simulink model "gps"  (Simulink 7.5)
settings: Solver=ode45  StartTime=0.0  StopTime=10.0  RelTol=1e-3
undefined symbols (not defined in the file or in its folder): magnitude, serial
libraries: dspsrcs4 x32, dspsigops x4, dsparch4 x3, dspstat3 x3, dspindex x3, instrumentlib x2, tiiqmathlib x1, dspxfrm3 x1
settings Model: Creator=sisa  LastModifiedBy=sisa

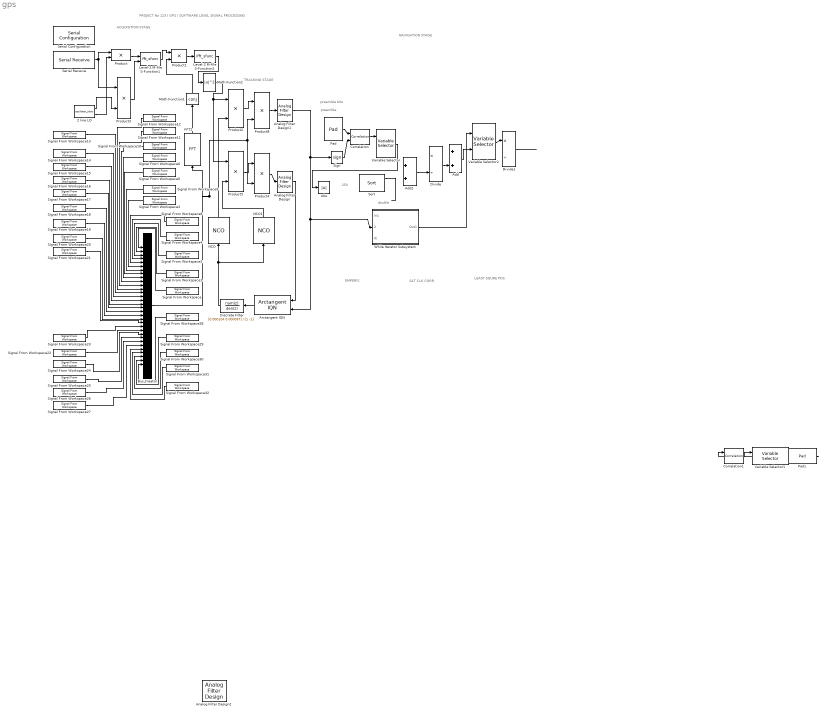
== system gps ==
  note: PROJECT No 123 ( GPS ) SOFTWARE LEVEL SIGNAL PROCESSING
  note: 253
  note: double
  note: preamble
  note: preamble bits
  note: ACQUISITION STAGE
  note: TRACKING STAGE
  note: EMPERIS
  note: NAVIGATION STAGE
  note: SAT CLK CORR
  note: LEAST SQURE POS
  2 line LO : M-S-Function  FunctionName=oscillator_sfunc  Parameters=1/38192000
  Abs : Abs  OutDataType=fixdt(1, 16)  OutScaling=2^0
  Add : Sum  OutDataType=fixdt(1, 16)  OutScaling=2^-10
  Add1 : Sum  OutDataType=fixdt(1, 16)  OutScaling=2^-10
  Analog Filter Design : dsparch4/Analog Filter Design  method=Butterworth  filttype=Lowpass  N=8  Wlo=30  Whi=80  Rp=2  Rs=40
  Analog Filter Design1 : dsparch4/Analog Filter Design  method=Chebyshev I  filttype=Lowpass  N=8  Wlo=30  Whi=80  Rp=2  Rs=40
  Analog Filter Design2 : dsparch4/Analog Filter Design  method=Butterworth  filttype=Lowpass  N=8  Wlo=30  Whi=80  Rp=2  Rs=40
  Arctangent IQN : tiiqmathlib/Arctangent IQN  tanOption=atan2PU (per unit)
  Bus Creator : BusCreator  Inputs=32  UseBusObject=on
  Correlation : dspstat3/Correlation  DialogController=dspDDGCreate  DialogControllerArgs=DataTag0  domain=Time  outputDataTypeStr=Inherit: Same as accumulator  outputLastDataTypeStr=Inherit: Same as accumulator  outputMin=[]  outputMax=[]  roundingMode=Floor  overflowMode=off
  Correlation1 : dspstat3/Correlation  DialogController=dspDDGCreate  DialogControllerArgs=DataTag1  domain=Time  outputDataTypeStr=Inherit: Same as accumulator  outputLastDataTypeStr=Inherit: Same as accumulator  outputMin=[]  outputMax=[]  roundingMode=Floor  overflowMode=off
  Discrete Filter : DiscreteFilter  Numerator=[0.000104 0.000097]  Denominator=[1 -1]  SampleTime=1
  Divide : Product  Inputs=*/  OutDataType=fixdt(1, 16)  OutScaling=2^-10
  Divide1 : Product  Inputs=*/  OutDataType=fixdt(1, 16)  OutScaling=2^-10
  FFT2 : dspxfrm3/FFT  DialogController=dspDDGCreate  DialogControllerArgs=DataTag2  CompMethod=Table lookup  TableOpt=NEW  TableOptActive=Speed  BitRevOrder=off  InheritFFTLength=on  FFTLength=64  SkipNorm=off  firstCoeffDataTypeStr=Inherit: Same word length as input  firstCoeffLastDataTypeStr=Inherit: Same word length as input  outputMin=[]  outputMax=[]  roundingMode=Floor  overflowMode=off
  Level-2 M-file S-Function1 : M-S-Function  FunctionName=fft_sfunc
  Level-2 M-file S-Function2 : M-S-Function  FunctionName=ifft_sfunc
  Math Function1 : Math  Operator=conj  OutputSignalType=complex  OutDataType=fixdt(1, 16)  OutScaling=2^0  SaturateOnIntegerOverflow=on
  Math Function2 : Math  Operator=magnitude^2  OutputSignalType=real  OutDataType=fixdt(1, 16)  OutScaling=2^0  SaturateOnIntegerOverflow=on
  NCO : dspsigops/NCO  DialogController=dspdialog.NCO  AccIncSrc=Input port  AccInc=100  PhaseOffsetSrc=Specify via dialog  PhaseOffset=0  AccumWL=16  HasDither=on  DitherWL=4  PNgeneratorLength=19  HasPhaseQuantizer=on  TableDepth=12  HasOutputPhaseError=off  Formula=Cosine  DataType=Binary point scaling  OutputWL=16  OutputFL=14  CompMethod=Table lookup (no interpolation)  SampleTime=1  SamplesPerFrame=1
  NCO1 : dspsigops/NCO  DialogController=dspdialog.NCO  AccIncSrc=Input port  AccInc=100  PhaseOffsetSrc=Specify via dialog  PhaseOffset=0  AccumWL=16  HasDither=on  DitherWL=4  PNgeneratorLength=19  HasPhaseQuantizer=on  TableDepth=12  HasOutputPhaseError=off  Formula=Sine  DataType=Binary point scaling  OutputWL=16  OutputFL=14  CompMethod=Table lookup (no interpolation)  SampleTime=1  SamplesPerFrame=1
  Pad : dspsigops/Pad  padAlong=Columns  dimsToPad=1  valSrc=Specify via dialog  padVal=0  spec=Output size  padNumOutRowsSpecMethod=User-specified  numOutRows=1  padNumOutColsSpecMethod=User-specified  numOutCols=1  isVarDimsMode=off  padBeginning=0  padEnd=0  outSizeMode=User-specified  outSize=1  padSigAt=End  trunc_flag=None  roundingMode=Floor  overflowMode=off  truncOrWrapMode=Truncate  wrap_flag=None
  Pad1 : dspsigops/Pad  padAlong=Columns  dimsToPad=1  valSrc=Specify via dialog  padVal=0  spec=Output size  padNumOutRowsSpecMethod=User-specified  numOutRows=1  padNumOutColsSpecMethod=User-specified  numOutCols=1  isVarDimsMode=off  padBeginning=0  padEnd=0  outSizeMode=User-specified  outSize=1  padSigAt=End  trunc_flag=None  roundingMode=Floor  overflowMode=off  truncOrWrapMode=Truncate  wrap_flag=None
  Product{,1..5,8} (7 alike) : Product  OutDataType=fixdt(1, 16)  OutScaling=2^0  RndMeth=Zero
  Serial Configuration : instrumentlib/Serial Configuration  Priority=-200000  DialogController=instrumentcreatedialog  DialogControllerArgs=DataTag3  ComPortMenu=COM1  ComPort=COM1  ObjConstructor=serial('COM1');  BaudRate=9600  DataBits=8  Parity=none  StopBits=1  FlowControl=none  Timeout=10  ByteOrder=LittleEndian
  Serial Receive : instrumentlib/Serial Receive  DialogController=instrumentcreatedialog  DialogControllerArgs=DataTag4  ComPortMenu=COM1  ComPort=COM1  ObjConstructor=serial('COM1');  Header=none  Terminator=<none>  DataSize="[1  1]"  DataType=uint8  EnableBlockingMode=on  ActionDataUnavailable=Output last received value  CustomValue=0  SampleTime=0.01
  Sign : Signum
  Signal From Workspace : dspsrcs4/Signal From Workspace  SystemSampleTime=-1  X=PN01  Ts=1  nsamps=1  OutputAfterFinalValue=Setting to zero  ignoreOrWarnInputAndFrameLengths=off
  Signal From Workspace1 : dspsrcs4/Signal From Workspace  SystemSampleTime=-1  X=PN02  Ts=1  nsamps=1  OutputAfterFinalValue=Setting to zero  ignoreOrWarnInputAndFrameLengths=off
  Signal From Workspace10 : dspsrcs4/Signal From Workspace  SystemSampleTime=-1  X=PN10  Ts=1  nsamps=1  OutputAfterFinalValue=Setting to zero  ignoreOrWarnInputAndFrameLengths=off
  Signal From Workspace11 : dspsrcs4/Signal From Workspace  SystemSampleTime=-1  X=PN11  Ts=1  nsamps=1  OutputAfterFinalValue=Setting to zero  ignoreOrWarnInputAndFrameLengths=off
  Signal From Workspace12 : dspsrcs4/Signal From Workspace  SystemSampleTime=-1  X=PN12  Ts=1  nsamps=1  OutputAfterFinalValue=Setting to zero  ignoreOrWarnInputAndFrameLengths=off
  Signal From Workspace13 : dspsrcs4/Signal From Workspace  SystemSampleTime=-1  X=PN13  Ts=1  nsamps=1  OutputAfterFinalValue=Setting to zero  ignoreOrWarnInputAndFrameLengths=off
  Signal From Workspace14 : dspsrcs4/Signal From Workspace  SystemSampleTime=-1  X=PN14  Ts=1  nsamps=1  OutputAfterFinalValue=Setting to zero  ignoreOrWarnInputAndFrameLengths=off
  Signal From Workspace15 : dspsrcs4/Signal From Workspace  SystemSampleTime=-1  X=PN15  Ts=1  nsamps=1  OutputAfterFinalValue=Setting to zero  ignoreOrWarnInputAndFrameLengths=off
  Signal From Workspace16 : dspsrcs4/Signal From Workspace  SystemSampleTime=-1  X=PN16  Ts=1  nsamps=1  OutputAfterFinalValue=Setting to zero  ignoreOrWarnInputAndFrameLengths=off
  Signal From Workspace17 : dspsrcs4/Signal From Workspace  SystemSampleTime=-1  X=PN17  Ts=1  nsamps=1  OutputAfterFinalValue=Setting to zero  ignoreOrWarnInputAndFrameLengths=off
  Signal From Workspace18 : dspsrcs4/Signal From Workspace  SystemSampleTime=-1  X=PN18  Ts=1  nsamps=1  OutputAfterFinalValue=Setting to zero  ignoreOrWarnInputAndFrameLengths=off
  Signal From Workspace19 : dspsrcs4/Signal From Workspace  SystemSampleTime=-1  X=PN19  Ts=1  nsamps=1  OutputAfterFinalValue=Setting to zero  ignoreOrWarnInputAndFrameLengths=off
  Signal From Workspace2 : dspsrcs4/Signal From Workspace  SystemSampleTime=-1  X=PN03  Ts=1  nsamps=1  OutputAfterFinalValue=Setting to zero  ignoreOrWarnInputAndFrameLengths=off
  Signal From Workspace20 : dspsrcs4/Signal From Workspace  SystemSampleTime=-1  X=PN20  Ts=1  nsamps=1  OutputAfterFinalValue=Setting to zero  ignoreOrWarnInputAndFrameLengths=off
  Signal From Workspace21 : dspsrcs4/Signal From Workspace  SystemSampleTime=-1  X=PN21  Ts=1  nsamps=1  OutputAfterFinalValue=Setting to zero  ignoreOrWarnInputAndFrameLengths=off
  Signal From Workspace22 : dspsrcs4/Signal From Workspace  SystemSampleTime=-1  X=PN23  Ts=1  nsamps=1  OutputAfterFinalValue=Setting to zero  ignoreOrWarnInputAndFrameLengths=off
  Signal From Workspace23 : dspsrcs4/Signal From Workspace  SystemSampleTime=-1  X=PN22  Ts=1  nsamps=1  OutputAfterFinalValue=Setting to zero  ignoreOrWarnInputAndFrameLengths=off
  Signal From Workspace24 : dspsrcs4/Signal From Workspace  SystemSampleTime=-1  X=PN24  Ts=1  nsamps=1  OutputAfterFinalValue=Setting to zero  ignoreOrWarnInputAndFrameLengths=off
  Signal From Workspace25 : dspsrcs4/Signal From Workspace  SystemSampleTime=-1  X=PN25  Ts=1  nsamps=1  OutputAfterFinalValue=Setting to zero  ignoreOrWarnInputAndFrameLengths=off
  Signal From Workspace26 : dspsrcs4/Signal From Workspace  SystemSampleTime=-1  X=PN26  Ts=1  nsamps=1  OutputAfterFinalValue=Setting to zero  ignoreOrWarnInputAndFrameLengths=off
  Signal From Workspace27 : dspsrcs4/Signal From Workspace  SystemSampleTime=-1  X=PN27  Ts=1  nsamps=1  OutputAfterFinalValue=Setting to zero  ignoreOrWarnInputAndFrameLengths=off
  Signal From Workspace28 : dspsrcs4/Signal From Workspace  SystemSampleTime=-1  X=PN28  Ts=1  nsamps=1  OutputAfterFinalValue=Setting to zero  ignoreOrWarnInputAndFrameLengths=off
  Signal From Workspace29 : dspsrcs4/Signal From Workspace  SystemSampleTime=-1  X=PN29  Ts=1  nsamps=1  OutputAfterFinalValue=Setting to zero  ignoreOrWarnInputAndFrameLengths=off
  Signal From Workspace3 : dspsrcs4/Signal From Workspace  SystemSampleTime=-1  X=PN06  Ts=1  nsamps=1  OutputAfterFinalValue=Setting to zero  ignoreOrWarnInputAndFrameLengths=off
  Signal From Workspace30 : dspsrcs4/Signal From Workspace  SystemSampleTime=-1  X=PN30  Ts=1  nsamps=1  OutputAfterFinalValue=Setting to zero  ignoreOrWarnInputAndFrameLengths=off
  Signal From Workspace31 : dspsrcs4/Signal From Workspace  SystemSampleTime=-1  X=PN31  Ts=1  nsamps=1  OutputAfterFinalValue=Setting to zero  ignoreOrWarnInputAndFrameLengths=off
  Signal From Workspace32 : dspsrcs4/Signal From Workspace  SystemSampleTime=-1  X=PN32  Ts=1  nsamps=1  OutputAfterFinalValue=Setting to zero  ignoreOrWarnInputAndFrameLengths=off
  Signal From Workspace4 : dspsrcs4/Signal From Workspace  SystemSampleTime=-1  X=PN04  Ts=1  nsamps=1  OutputAfterFinalValue=Setting to zero  ignoreOrWarnInputAndFrameLengths=off
  Signal From Workspace5 : dspsrcs4/Signal From Workspace  SystemSampleTime=-1  X=PN08  Ts=1  nsamps=1  OutputAfterFinalValue=Setting to zero  ignoreOrWarnInputAndFrameLengths=off
  Signal From Workspace6 : dspsrcs4/Signal From Workspace  SystemSampleTime=-1  X=PN09  Ts=1  nsamps=1  OutputAfterFinalValue=Setting to zero  ignoreOrWarnInputAndFrameLengths=off
  Signal From Workspace8 : dspsrcs4/Signal From Workspace  SystemSampleTime=-1  X=PN05  Ts=1  nsamps=1  OutputAfterFinalValue=Setting to zero  ignoreOrWarnInputAndFrameLengths=off
  Signal From Workspace9 : dspsrcs4/Signal From Workspace  SystemSampleTime=-1  X=PN07  Ts=1  nsamps=1  OutputAfterFinalValue=Setting to zero  ignoreOrWarnInputAndFrameLengths=off
  Sort : dspstat3/Sort  DialogController=dspDDGCreate  DialogControllerArgs=DataTag5  otype=Value and Index  dir=Ascending  sortAlg=Quick sort  accumDataTypeStr=Inherit: Same as product output  accumLastDataTypeStr=Inherit: Same as product output  roundingMode=Floor  overflowMode=off
  Variable Selector : dspindex/Variable Selector  NumInputs=1  rowsOrCols=Rows  IdxMode=Variable  Elements=[1 3]  ZerOneIdxMode=Zero-based  errmode=Clip and Warn  FillMode=on  FillValues=0
  Variable Selector1 : dspindex/Variable Selector  NumInputs=1  rowsOrCols=Rows  IdxMode=Variable  Elements=[1 3]  ZerOneIdxMode=Zero-based  errmode=Clip and Warn  FillMode=on  FillValues=0
  Variable Selector2 : dspindex/Variable Selector  NumInputs=1  rowsOrCols=Rows  IdxMode=Variable  Elements=[1 3]  ZerOneIdxMode=One-based  errmode=Clip Index  FillMode=on  FillValues=0
  While Iterator Subsystem : Subsystem  TreatAsAtomicUnit=on
  wires:
  Serial Receive/1 -> Product/1, Product3/1
  FFT2/1 -> Math Function1/1
  Product3/1 -> Level-2 M-file S-Function1/2
  Level-2 M-file S-Function2/1 -> Math Function2/1
  2 line LO/1 -> Product3/2
  2 line LO/2 -> Product/2
  Bus Creator/1 -> FFT2/1, Product8/2, Product4/2
  Signal From Workspace/1 -> Bus Creator/1
  Signal From Workspace1/1 -> Bus Creator/2
  Signal From Workspace4/1 -> Bus Creator/4
  Signal From Workspace2/1 -> Bus Creator/3
  Signal From Workspace8/1 -> Bus Creator/5
  Signal From Workspace3/1 -> Bus Creator/6
  Signal From Workspace9/1 -> Bus Creator/7
  Signal From Workspace5/1 -> Bus Creator/8
  Signal From Workspace6/1 -> Bus Creator/9
  Signal From Workspace10/1 -> Bus Creator/10
  Signal From Workspace11/1 -> Bus Creator/11
  Signal From Workspace12/1 -> Bus Creator/12
  Signal From Workspace13/1 -> Bus Creator/13
  Signal From Workspace14/1 -> Bus Creator/14
  Signal From Workspace15/1 -> Bus Creator/15
  Signal From Workspace16/1 -> Bus Creator/16
  Signal From Workspace17/1 -> Bus Creator/17
  Signal From Workspace18/1 -> Bus Creator/18
  Signal From Workspace19/1 -> Bus Creator/19
  Signal From Workspace28/1 -> Bus Creator/32
  Signal From Workspace32/1 -> Bus Creator/28
  Signal From Workspace20/1 -> Bus Creator/20
  Signal From Workspace21/1 -> Bus Creator/21
  Signal From Workspace23/1 -> Bus Creator/22
  Signal From Workspace22/1 -> Bus Creator/23
  Signal From Workspace24/1 -> Bus Creator/24
  Signal From Workspace25/1 -> Bus Creator/25
  Signal From Workspace26/1 -> Bus Creator/26
  Signal From Workspace27/1 -> Bus Creator/27
  NCO/1 -> Product2/2
  Product5/1 -> Product4/1
  Product4/1 -> Analog Filter Design/1
  Product8/1 -> Analog Filter Design1/1
  Product2/1 -> Product8/1
  Analog Filter Design/1 -> Arctangent IQN/1
  Analog Filter Design1/1 -> Sign/1, Arctangent IQN/2, While Iterator Subsystem/2
  NCO1/1 -> Product5/2
  Signal From Workspace29/1 -> Bus Creator/31
  Signal From Workspace30/1 -> Bus Creator/30
  Signal From Workspace31/1 -> Bus Creator/29
  Product1/1 -> Level-2 M-file S-Function2/1
  Pad1/1 -> Correlation1/1
  ? -> Correlation1/2
  Correlation1/1 -> Variable Selector1/1
  Pad/1 -> Correlation/1
  Sign/1 -> Correlation/2
  Correlation/1 -> Variable Selector/1
  Variable Selector/1 -> Abs/1
  ? -> Sort/1
  Sort/1 -> ?
  Math Function2/1 -> Product5/1, Product2/1
  ? -> While Iterator Subsystem/1(In1)
  Add/1 -> Variable Selector2/2
  Add1/1 -> Divide/2
  Divide/1 -> Add/2
  Variable Selector2/1 -> Divide1/1
  Divide1/1 -> ?
  While Iterator Subsystem/1(Out1) -> Variable Selector2/1
  Arctangent IQN/1 -> Discrete Filter/1
  Discrete Filter/1 -> NCO/1, NCO1/1
  Math Function1/1 -> Product1/2
  Level-2 M-file S-Function1/1 -> Product1/1
  Product/1 -> Level-2 M-file S-Function1/1

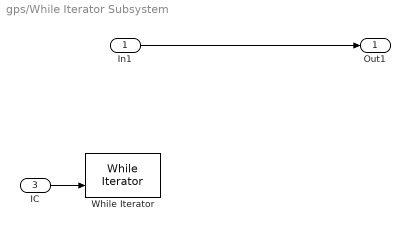
== system gps/While Iterator Subsystem ==
  In1 : Inport  OutDataType=fixdt(1, 16)  OutScaling=2^0
  IC : Inport  Port=3  OutDataType=fixdt(1, 16)  OutScaling=2^0
  While Iterator : WhileIterator  ShowIterationPort=on
  Out1 : Outport  OutDataType=fixdt(1, 16)  OutScaling=2^0
  wires:
  IC/1 -> While Iterator/2
  In1/1 -> Out1/1
